simulink model "pendul_sim"  (R2015a)
settings: Solver=ode45  StartTime=0.0  StopTime=4  RelTol=1e-3
values from neighbouring files (symbols this model uses):
  m = 0.700    (= 0.7)    [pendul.m]
  S = 0    [pendul.m]    (also in pendul2.m)
  sensor_den = [Lf*Cf (Rf+R0)*Cf 1]    [pendul.m]
  sensor_num = [R0*Cf 0]    [pendul.m]
  system_den = [m_v*L 0 -m*g]    [pendul.m]
  system_num = [1]    [pendul.m]
  vogn = 1.355    [pendul.m]    (also in pendul2.m = 1.37)
  vogn_offset = 0.655    [pendul.m]
libraries: simulink x1
settings Model: Creator=jorn  LastModifiedBy=jorn

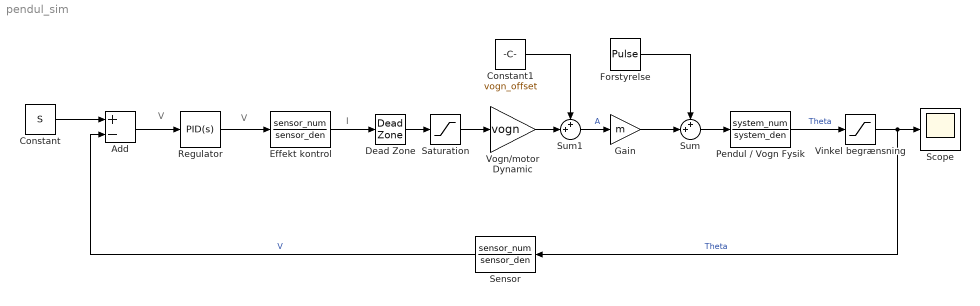
== system pendul_sim ==
  note: I
  note: V
  note: V
  Add : Sum  Inputs=+-
  Constant : Constant  Value=S
  Constant1 : Constant  Value=vogn_offset
  Dead Zone : DeadZone  LowerValue=-1  UpperValue=1  SaturateOnIntegerOverflow=on
  Effekt kontrol : TransferFcn  Numerator=sensor_num  Denominator=sensor_den
  Forstyrelse : DiscretePulseGenerator  PulseType=Time based  Period=10  PulseWidth=0.01  PhaseDelay=1
  Gain : Gain  Gain=m
  Pendul / Vogn Fysik : TransferFcn  Numerator=system_num  Denominator=system_den
  Regulator : simulink/Continuous/PID Controller  Controller=PID  TimeDomain=Continuous-time  SampleTime=-1  IntegratorMethod=Forward Euler  FilterMethod=Forward Euler  Form=Parallel  UseFilter=on  ControllerParametersSource=internal  P=1  I=1  D=0  N=100  InitialConditionSource=internal  InitialConditionForIntegrator=0  InitialConditionForFilter=0  ExternalReset=none  LimitOutput=off  UpperSaturationLimit=inf  LowerSaturationLimit=-inf  LinearizeAsGain=on  AntiWindupMode=none  Kb=1  TrackingMode=off  Kt=1  PParamMin=[]  PParamMax=[]  IParamMin=[]  IParamMax=[]  DParamMin=[]  DParamMax=[]  NParamMin=[]  NParamMax=[]  KbParamMin=[]  KbParamMax=[]  KtParamMin=[]  KtParamMax=[]  POutMin=[]  POutMax=[]  IOutMin=[]  IOutMax=[]  DOutMin=[]  DOutMax=[]  NOutMin=[]  NOutMax=[]  KbOutMin=[]  KbOutMax=[]  KtOutMin=[]  KtOutMax=[]  IntegratorOutMin=[]  IntegratorOutMax=[]  FilterOutMin=[]  FilterOutMax=[]  SumOutMin=[]  SumOutMax=[]  SumI1OutMin=[]  SumI1OutMax=[]  SumI2OutMin=[]  SumI2OutMax=[]  SumI3OutMin=[]  SumI3OutMax=[]  SumDOutMin=[]  SumDOutMax=[]  SaturationOutMin=[]  SaturationOutMax=[]  IntegratorContinuousStateAttributes=''  IntegratorStateMustResolveToSignalObject=off  IntegratorRTWStateStorageClass=Auto  FilterContinuousStateAttributes=''  FilterStateMustResolveToSignalObject=off  FilterRTWStateStorageClass=Auto  DifferentiatorICPrevScaledInput=0  DifferentiatorOutMin=[]  DifferentiatorOutMax=[]
  Saturation : Saturate  UpperLimit=2.5  LowerLimit=-2.5
  Scope : Scope
      settings: TimeRange=1.2  YMin=-0.9  YMax=0  ScrollMode=on
  Sensor : TransferFcn  Numerator=sensor_num  Denominator=sensor_den
  Sum : Sum  Inputs=++|
  Sum1 : Sum  Inputs=++|
  Vinkel begrænsning : Saturate  UpperLimit=45  LowerLimit=-45
  Vogn/motor Dynamic : Gain  Gain=vogn
  wires:
  Sensor/1 -> Add/2  "V"
  Constant/1 -> Add/1
  Sum/1 -> Pendul / Vogn Fysik/1
  Forstyrelse/1 -> Sum/1
  Gain/1 -> Sum/2
  Constant1/1 -> Sum1/1
  Sum1/1 -> Gain/1  "A"
  Pendul / Vogn Fysik/1 -> Vinkel begrænsning/1  "Theta"
  Vinkel begrænsning/1 -> Scope/1, Sensor/1  "Theta"
  Vogn/motor Dynamic/1 -> Sum1/2
  Dead Zone/1 -> Saturation/1
  Saturation/1 -> Vogn/motor Dynamic/1
  Effekt kontrol/1 -> Dead Zone/1
  Add/1 -> Regulator/1
  Regulator/1 -> Effekt kontrol/1
